simulink model "arduinoModel"  (R2023b)
settings: Solver=FixedStepAuto  StartTime=0.0  StopTime=inf  RelTol=1e-3
libraries: arduinolib x3, simulink x1
settings Model: ExtModeTrigDuration=2  Creator=guido  LastModifiedBy=guido
settings OptimizationCC: EnhancedBackFolding=on  PassReuseOutputArgsAs=Individual arguments  ZeroExternalMemoryAtStartup=off  ZeroInternalMemoryAtStartup=off  MaxStackSize=64  OptimizeBlockOrder=speed  DifferentSizesBufferReuse=on  OptimizationCustomize=off  EfficientTunableParamExpr=on
settings DebuggingCC: ParameterTunabilityLossMsg=error
settings HardwareCC: ProdBitPerInt=16  ProdBitPerPointer=16  ProdBitPerSizeT=16  ProdBitPerPtrDiffT=16  ProdLargestAtomicFloat=None  ProdWordSize=8  ProdHWDeviceType=Atmel->AVR  UseEmbeddedCoderFeatures=off  UseSimulinkCoderFeatures=off
settings SFSimCC: MATLABDynamicMemAlloc=off
settings RTWCC: Description=Embedded Coder  SystemTargetFile=ert.tlc  HardwareBoard=Arduino Uno  TemplateMakefile=ert_default_tmf  Toolchain=Arduino AVR  BuildConfiguration=Faster Runs
settings CodeAppCC: ForceParamTrailComments=on  IgnoreCustomStorageClasses=off  OperatorAnnotations=on  SimulinkDataObjDesc=on  SFDataObjDesc=on  InsertBlockDesc=on
settings ERTTargetCC: SupportContinuousTime=on  SupportNonInlinedSFcns=on  SupportVariableSizeSignals=on  ExtModeTransport=3  ExtModeStaticAlloc=on  ExtModeAutomaticAllocSize=off  ExtModeStaticAllocSize=250  ExtModeMexFile=ext_xcp  ExtModeIntrfLevel=Level2 - Open

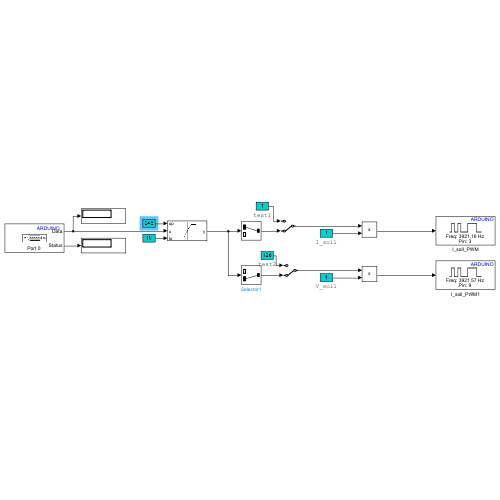
[thumbnail: Simulink's stored preview of the top-level diagram]
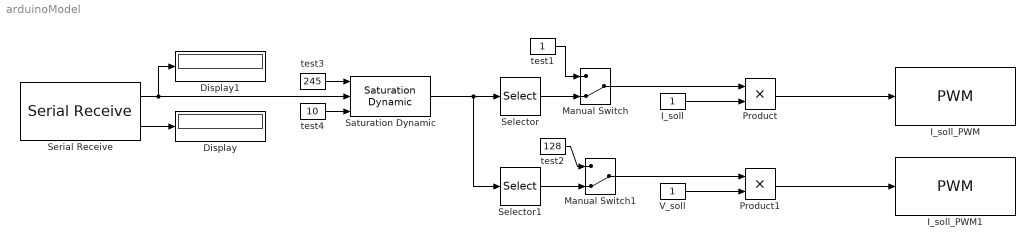
== system arduinoModel ==
  Display : Display
  Display1 : Display
  I_soll : Constant
  I_soll_PWM : arduinolib/PWM  pinNumber=3  frequencyType=Specify  desiredFrequency=3921.16  achievableFrequency=3921.16
  I_soll_PWM1 : arduinolib/PWM  pinNumber=9  frequencyType=Specify  desiredFrequency=3921.16  achievableFrequency=3921.5686
  Manual Switch : ManualSwitch  CurrentSetting=0
  Manual Switch1 : ManualSwitch  CurrentSetting=0
  Product : Product
  Product1 : Product
  Saturation Dynamic : simulink/Discontinuities/Saturation Dynamic  OutMin=[]  OutMax=[]  OutDataTypeStr=Inherit: Same as second input  OutDataType=fixdt(1, 16)  OutScaling=2^-10  DoSatur=off
  Selector : Selector  InputPortWidth=2  IndexOptions=Index vector (dialog)  Indices=[1]  OutputSizes=1
  Selector1 : Selector  InputPortWidth=2  IndexOptions=Index vector (dialog)  Indices=[2]  OutputSizes=1
  Serial Receive : arduinolib/Serial Receive  isARMArch=off  portNumber=0  DataType=uint16  Datalength=2  SampleTime=0.1  showOutStatus=on  blockPlatform=arduino
  V_soll : Constant
  test1 : Constant
  test2 : Constant  Value=128
  test3 : Constant  Value=245
  test4 : Constant  Value=10
  wires:
  Product1/1 -> I_soll_PWM1/1
  I_soll/1 -> Product/2
  V_soll/1 -> Product1/2
  Serial Receive/2 -> Display/1
  Selector/1 -> Manual Switch/2
  Serial Receive/1 -> Saturation Dynamic/2, Display1/1
  Product/1 -> I_soll_PWM/1
  Manual Switch/1 -> Product/1
  Selector1/1 -> Manual Switch1/2
  Manual Switch1/1 -> Product1/1
  test1/1 -> Manual Switch/1
  test2/1 -> Manual Switch1/1
  Saturation Dynamic/1 -> Selector1/1, Selector/1
  test3/1 -> Saturation Dynamic/1
  test4/1 -> Saturation Dynamic/3
